simulink model "test_fastterminal_formation_gazebo_paper_cts23a"  (R2023a)
settings: Solver=FixedStepAuto  StartTime=0.0  StopTime=inf  RelTol=1e-3
undefined symbols (not defined in the file or in its folder): angular, DiscIntNeverNeededParam, linear
libraries: ros2lib x11, simulink x4, robotcorelib x4
(part 1 of 2)
settings Model: Creator=johvany  LastModifiedBy=l15
settings OptimizationCC: EnhancedBackFolding=on  PassReuseOutputArgsThreshold=0  MaxStackSize=64  OptimizeBlockOrder=speed  DifferentSizesBufferReuse=on  OptimizationCustomize=off
settings DebuggingCC: ParameterTunabilityLossMsg=error
settings HardwareCC: ProdBitPerLong=64  ProdHWDeviceType=Intel->x86-64 (Linux 64)  UseEmbeddedCoderFeatures=off
settings SFSimCC: MATLABDynamicMemAlloc=off
settings RTWCC: Description=Simulink Desktop Real-Time  SystemTargetFile=sldrt.tlc  TemplateMakefile=sldrt.tmf  Toolchain=Colcon Tools  RTWCompilerOptimization=on
settings CodeAppCC: ForceParamTrailComments=on  MaxIdLength=95  OperatorAnnotations=on
settings SimulinkDesktopRealTimeCC: TargetLibSuffix=_sldrt.a  TargetPreCompLibLocation=/usr/local/MATLAB/R2023b/toolbox/sldrt/lib/glnxa64  TargetLangStandard=C89/C90 (ANSI)

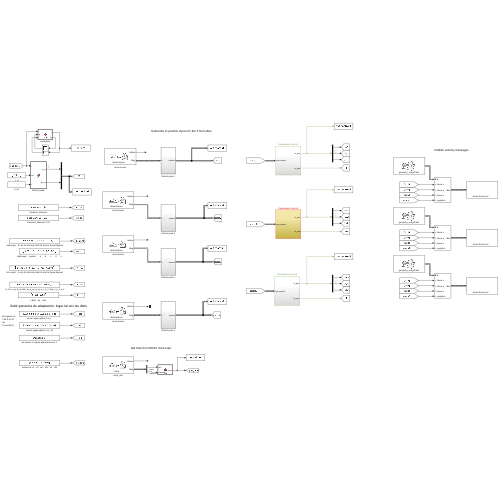
[thumbnail: Simulink's stored preview of the top-level diagram]
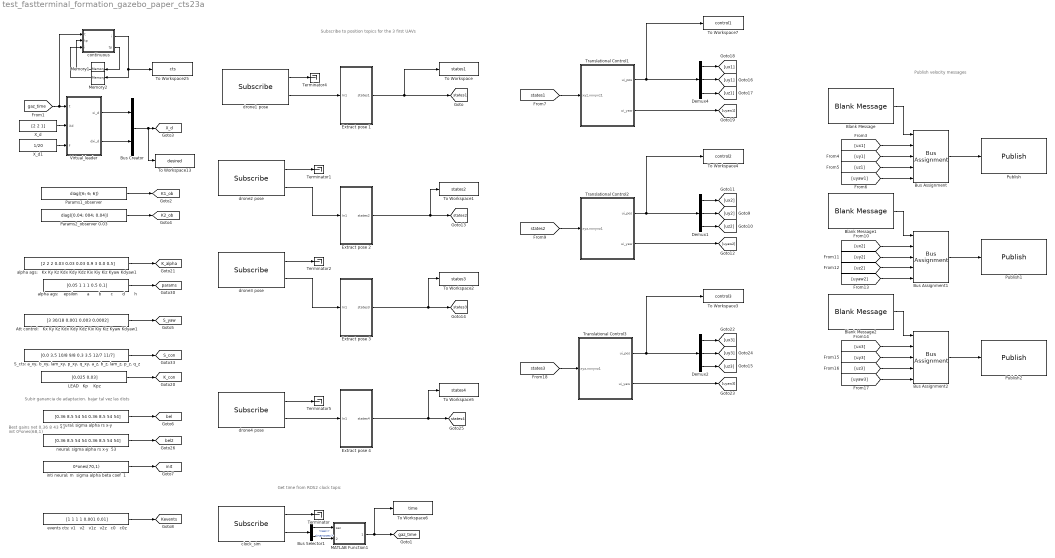
== system test_fastterminal_formation_gazebo_paper_cts23a ==
  note: Subir ganancia de adaptacion. bajar tal vez las dists
  note: Publish velocity messages
  note: Subscribe to position topics for the 3 first UAVs
  note: Get time from ROS2 clock topic
  note: Best gains net
      | 0.36 8 43 43
      | init
      | 0*ones(68,1)
  Att control:   Kx Ky Kz Kdx Kdy Kdz Kix Kiy Kiz Kyaw Kdyaw1 : Constant  Value=[3 30/18 0.001 0.003 0.0002]
  Blank Message : ros2lib/Blank Message  messageClass=Message  entityType=geometry_msgs/Twist  messageType=geometry_msgs/Twist  SampleTime=inf
  Blank Message1 : ros2lib/Blank Message  messageClass=Message  entityType=geometry_msgs/Twist  messageType=geometry_msgs/Twist  SampleTime=inf
  Blank Message2 : ros2lib/Blank Message  messageClass=Message  entityType=geometry_msgs/Twist  messageType=geometry_msgs/Twist  SampleTime=inf
  Bus Assignment : BusAssignment  AssignedSignals=linear.x,linear.y,linear.z,angular.z
  Bus Assignment1 : BusAssignment  AssignedSignals=linear.x,linear.y,linear.z,angular.z
  Bus Assignment2 : BusAssignment  AssignedSignals=linear.x,linear.y,linear.z,angular.z
  Bus Creator : BusCreator  Inputs=2
  Bus Selector1 : BusSelector  OutputSignals=clock.sec,clock.nanosec
  Demux1 : Demux  Outputs=3
  Demux2 : Demux  Outputs=3
  Demux4 : Demux  Outputs=3
  Extract pose 1 : Subsystem
  Extract pose 2 : Subsystem
  Extract pose 3 : Subsystem
  Extract pose 4 : Subsystem
  LEAD   Kp    Kpz : Constant  Value=[0.025 0.03]
  MATLAB Function1 : MATLAB Function  TreatAsAtomicUnit=on
  Memory1 : Memory
  Memory2 : Memory
  Params1_observer : Constant  Value=diag([6; 6; 6])
  Params2_observer 0.03 : Constant  Value=diag([0.04; 004; 0.04])
  Publish : ros2lib/Publish  topicSource=Select from ROS network  topic=/drone1/cmd_vel  messageType=geometry_msgs/Twist  QOSHistory=Keep last  QOSDepth=1  QOSReliability=Reliable  QOSDurability=Volatile
  Publish1 : ros2lib/Publish  topicSource=Select from ROS network  topic=/drone2/cmd_vel  messageType=geometry_msgs/Twist  QOSHistory=Keep last  QOSDepth=1  QOSReliability=Reliable  QOSDurability=Volatile
  Publish2 : ros2lib/Publish  topicSource=Select from ROS network  topic=/drone3/cmd_vel  messageType=geometry_msgs/Twist  QOSHistory=Keep last  QOSDepth=1  QOSReliability=Reliable  QOSDurability=Volatile
  "S_cts: a_xy, b_xy, lam_xy, p_xy, q_xy, a_z, b_z, lam_z, p_z, q_z" : Constant  Value=[0.0 3.5 10/8 9/8 0.3 3.5 12/7 11/7]
  Terminator{,1..2,4..5} (5 alike) : Terminator
  To Workspace : ToWorkspace  VariableName=states1  SampleTime=-1
  To Workspace1 : ToWorkspace  VariableName=states2  SampleTime=-1
  To Workspace13 : ToWorkspace  VariableName=desired  SampleTime=-1
  To Workspace2 : ToWorkspace  VariableName=states3  SampleTime=-1
  To Workspace25 : ToWorkspace  VariableName=cts  SampleTime=-1
  To Workspace3 : ToWorkspace  VariableName=control3  SampleTime=-1
  To Workspace4 : ToWorkspace  VariableName=control2  SampleTime=-1
  To Workspace5 : ToWorkspace  VariableName=states4  SampleTime=-1
  To Workspace6 : ToWorkspace  VariableName=time  SampleTime=-1
  To Workspace7 : ToWorkspace  VariableName=control1  SampleTime=-1
  Translational Control1 : Subsystem
  Translational Control2 : Subsystem
  Translational Control3 : Subsystem
  Virtual_leader : MATLAB Function  TreatAsAtomicUnit=on
  X_d : Constant  Value=[2 2 1]
  X_d1 : Constant  Value=1/20
  alpha ags:    epsilon       a       b       c       d       h : Constant  Value=[0.05 1 1 1 0.5 0.1]
  alpha ags:   Kx Ky Kz Kdx Kdy Kdz Kix Kiy Kiz Kyaw Kdyaw1 : Constant  Value=[2 2 2 0.03 0.03 0.03 0.9 3 0.0 0.5]
  clock_sim : ros2lib/Subscribe  topicSource=Select from ROS network  topic=/clock  messageType=rosgraph_msgs/Clock  sampleTime=-1  QOSHistory=Keep last  QOSDepth=1  QOSReliability=Reliable  QOSDurability=Volatile
  continuous : MATLAB Function  TreatAsAtomicUnit=on
  drone1 pose : ros2lib/Subscribe  topicSource=Select from ROS network  topic=/drone1/pose  messageType=geometry_msgs/PoseStamped  sampleTime=-1  QOSHistory=Keep last  QOSDepth=1  QOSReliability=Reliable  QOSDurability=Volatile
  drone2 pose : ros2lib/Subscribe  topicSource=Select from ROS network  topic=/drone2/pose  messageType=geometry_msgs/PoseStamped  sampleTime=-1  QOSHistory=Keep last  QOSDepth=1  QOSReliability=Reliable  QOSDurability=Volatile
  drone3 pose : ros2lib/Subscribe  topicSource=Select from ROS network  topic=/drone3/pose  messageType=geometry_msgs/PoseStamped  sampleTime=-1  QOSHistory=Keep last  QOSDepth=1  QOSReliability=Reliable  QOSDurability=Volatile
  drone4 pose : ros2lib/Subscribe  topicSource=Select from ROS network  topic=/drone4/pose  messageType=geometry_msgs/PoseStamped  sampleTime=-1  QOSHistory=Keep last  QOSDepth=1  QOSReliability=Reliable  QOSDurability=Volatile
  events cts: v1   v2   v1z   v2z   c0   c0z : Constant  Value=[1 1 1 1 0.001 0.01]
  inti neural: m  sigma alpha beta coef  1 : Constant  Value=0*ones(70,1)
  "neural: sigma alpha rs x-y  " : Constant  Value=[0.36 8.5 54 54 0.36 8.5 54 54]
  neural: sigma alpha rs x-y  53 : Constant  Value=[0.36 8.5 54 54 0.36 8.5 54 54]
  tag scope: K1_ob=global, K2_ob=global, K_alpha=global, K_con=global, Kevents=global, S_con=global, S_yaw=global, X_d=global, bel2=global, bel=global, gaz_time=global, init=global, params=global, states1=global, states2=global, states3=global, states4=global
  wires:
  clock_sim/1 -> Terminator/1
  drone2 pose/2 -> Extract pose 2/1(In1)
  drone2 pose/1 -> Terminator1/1
  drone3 pose/2 -> Extract pose 3/1(In1)
  drone3 pose/1 -> Terminator2/1
  Blank Message/1 -> Bus Assignment/1
  Bus Assignment/1 -> Publish/1
  Blank Message1/1 -> Bus Assignment1/1
  Bus Assignment1/1 -> Publish1/1
  Blank Message2/1 -> Bus Assignment2/1
  Bus Assignment2/1 -> Publish2/1
  clock_sim/2 -> Bus Selector1/1
  Bus Selector1/1 -> MATLAB Function1/1(sec)  "<sec>"
  Bus Selector1/2 -> MATLAB Function1/2(nanosec)  "<nanosec>"
  Virtual_leader/2(dxi_d) -> Bus Creator/2
  Bus Creator/1 -> To Workspace13/1, [X_d]
  Virtual_leader/1(xi_d) -> Bus Creator/1
  drone1 pose/1 -> Terminator4/1
  drone1 pose/2 -> Extract pose 1/1(In1)
  MATLAB Function1/1(gaz_time) -> To Workspace6/1, [gaz_time]
  Extract pose 1/1(states1) -> To Workspace/1, [states1]
  [ux1] -> Bus Assignment/2
  [uy1] -> Bus Assignment/3
  [uz1] -> Bus Assignment/4
  [uyaw1] -> Bus Assignment/5
  X_d/1 -> Virtual_leader/2(Xd)
  Extract pose 2/1(states2) -> To Workspace1/1, [states2]
  Extract pose 3/1(states3) -> To Workspace2/1, [states3]
  [ux2] -> Bus Assignment1/2
  [uy2] -> Bus Assignment1/3
  [uz2] -> Bus Assignment1/4
  [uyaw2] -> Bus Assignment1/5
  [uy3] -> Bus Assignment2/3
  [uyaw3] -> Bus Assignment2/5
  [uz3] -> Bus Assignment2/4
  [ux3] -> Bus Assignment2/2
  Translational Control1/2(ui_yaw) -> [uyaw1]
  Demux4/2 -> [uy1]
  Demux4/3 -> [uz1]
  [states1] -> Translational Control1/1(xyz,vxvyvz1)
  Demux4/1 -> [ux1]
  LEAD   Kp    Kpz/1 -> [K_con]
  alpha ags:   Kx Ky Kz Kdx Kdy Kdz Kix Kiy Kiz Kyaw Kdyaw1/1 -> [K_alpha]
  alpha ags:    epsilon       a       b       c       d       h/1 -> [params]
  X_d1/1 -> Virtual_leader/3(f)
  "S_cts: a_xy, b_xy, lam_xy, p_xy, q_xy, a_z, b_z, lam_z, p_z, q_z"/1 -> [S_con]
  "neural: sigma alpha rs x-y  "/1 -> [bel]
  inti neural: m  sigma alpha beta coef  1/1 -> [init]
  Translational Control1/1(ui_pos) -> Demux4/1, To Workspace7/1
  Params1_observer/1 -> [K1_ob]
  Params2_observer 0.03/1 -> [K2_ob]
  events cts: v1   v2   v1z   v2z   c0   c0z/1 -> [Kevents]
  Translational Control2/1(ui_pos) -> Demux1/1, To Workspace4/1
  Demux1/1 -> [ux2]
  [states2] -> Translational Control2/1(xyz,vxvyvz1)
  Demux1/3 -> [uz2]
  Demux1/2 -> [uy2]
  Translational Control2/2(ui_yaw) -> [uyaw2]
  Translational Control3/2(ui_yaw) -> [uyaw3]
  Demux2/2 -> [uy3]
  Demux2/3 -> [uz3]
  [states3] -> Translational Control3/1(xyz,vxvyvz1)
  Demux2/1 -> [ux3]
  Translational Control3/1(ui_pos) -> Demux2/1, To Workspace3/1
  Extract pose 4/1(states4) -> [states4], To Workspace5/1
  drone4 pose/1 -> Terminator5/1
  drone4 pose/2 -> Extract pose 4/1(In1)
  neural: sigma alpha rs x-y  53/1 -> [bel2]
  Memory1/1 -> continuous/2("tp ")
  Memory2/1 -> continuous/3("i ")
  [gaz_time] -> continuous/1(t), Virtual_leader/1(t)
  continuous/1(i) -> To Workspace25/1, Memory2/1
  continuous/2(tp) -> Memory1/1
  Att control:   Kx Ky Kz Kdx Kdy Kdz Kix Kiy Kiz Kyaw Kdyaw1/1 -> [S_yaw]

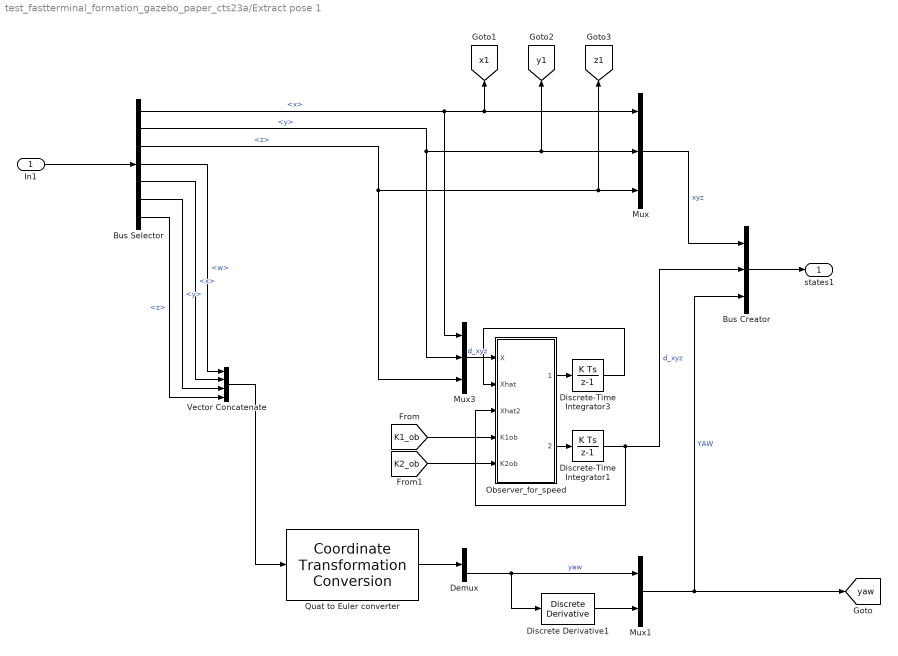
== system test_fastterminal_formation_gazebo_paper_cts23a/Extract pose 1 ==
  In1 : Inport
  Bus Creator : BusCreator  Inputs=3
  Bus Selector : BusSelector  OutputSignals=pose.position.x,pose.position.y,pose.position.z,pose.orientation.w,pose.orientation.x,pose.orientation.y,pose.orientation.z
  Demux : Demux  Outputs=3
  Discrete Derivative1 : simulink/Discrete/Discrete Derivative  gainval=1.0  ICPrevScaledInput=0.0  OutMin=[]  OutMax=[]  OutDataType=fixdt(1, 16)  OutScaling=2^-10  DoSatur=off
  Discrete-Time Integrator1 : DiscreteIntegrator  SampleTime=-1  UpperSaturationLimit=1  LowerSaturationLimit=-1  ICPrevOutput=DiscIntNeverNeededParam  ICPrevScaledInput=DiscIntNeverNeededParam
  Discrete-Time Integrator3 : DiscreteIntegrator  SampleTime=-1  UpperSaturationLimit=1  LowerSaturationLimit=-1  ICPrevOutput=DiscIntNeverNeededParam  ICPrevScaledInput=DiscIntNeverNeededParam
  Mux : Mux  Inputs=3
  Mux1 : Mux  Inputs=2
  Mux3 : Mux  Inputs=3
  Observer_for_speed : MATLAB Function  TreatAsAtomicUnit=on
  Quat to Euler converter : robotcorelib/Coordinate Transformation Conversion  InputRepresentation=Quaternion  InputEulerSequence=ZYX  ShowTrVecInputPort=on  OutputRepresentation=Euler Angles  OutputEulerSequence=XYZ  ShowTrVecOutputPort=on  SimulateUsing=Interpreted execution
      settings: LibrarySourceBlock=roslib/Utilities/Coordinate Transformation Conversion
  Vector Concatenate : Concatenate  NumInputs=4
  states1 : Outport
  tag scope: x1=global, y1=global, yaw=global, z1=global
  wires:
  Bus Selector/5 -> Vector Concatenate/2  "<x>"
  Quat to Euler converter/1 -> Demux/1
  Bus Selector/6 -> Vector Concatenate/3  "<y>"
  Bus Selector/7 -> Vector Concatenate/4  "<z>"
  Vector Concatenate/1 -> Quat to Euler converter/1
  In1/1 -> Bus Selector/1
  Bus Selector/4 -> Vector Concatenate/1  "<w>"
  Demux/3 -> Discrete Derivative1/1, Mux1/1  "yaw"
  Mux/1 -> Bus Creator/1  "xyz"
  Bus Creator/1 -> states1/1
  Discrete Derivative1/1 -> Mux1/2
  Bus Selector/3 -> Mux3/3, [z1], Mux/3  "<z>"
  Bus Selector/2 -> Mux3/2, [y1], Mux/2  "<y>"
  Bus Selector/1 -> Mux3/1, [x1], Mux/1  "<x>"
  Mux1/1 -> [yaw], Bus Creator/3  "YAW"
  Discrete-Time Integrator1/1 -> Observer_for_speed/3(Xhat2), Bus Creator/2  "d_xyz"
  Discrete-Time Integrator3/1 -> Observer_for_speed/2(Xhat)
  Observer_for_speed/1(dXhat_1) -> Discrete-Time Integrator3/1
  Observer_for_speed/2(dXhat_2) -> Discrete-Time Integrator1/1
  Mux3/1 -> Observer_for_speed/1(X)  "d_xyz"
  [K1_ob] -> Observer_for_speed/4(K1ob)
  [K2_ob] -> Observer_for_speed/5(K2ob)

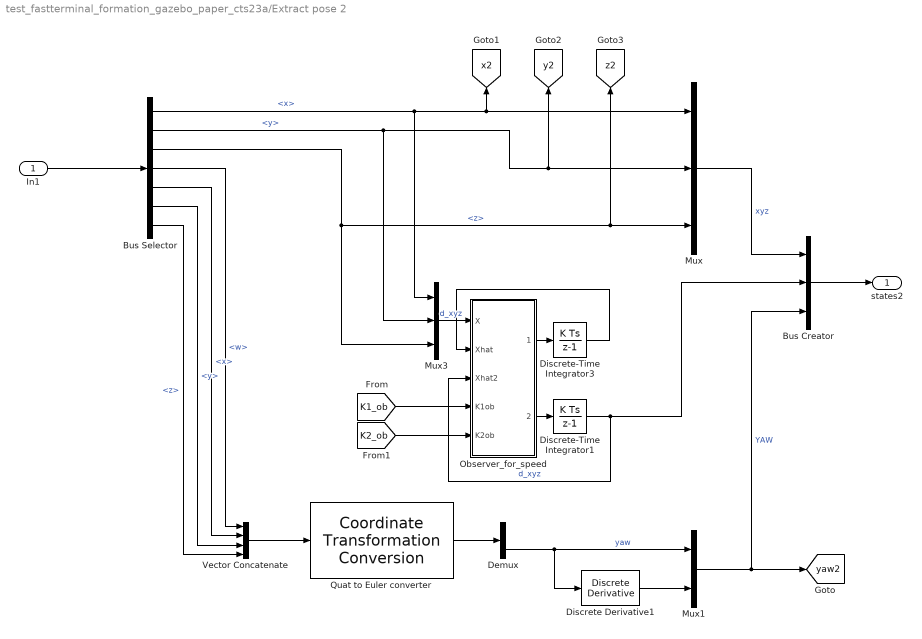
== system test_fastterminal_formation_gazebo_paper_cts23a/Extract pose 2 ==
  In1 : Inport
  Bus Creator : BusCreator  Inputs=3
  Bus Selector : BusSelector  OutputSignals=pose.position.x,pose.position.y,pose.position.z,pose.orientation.w,pose.orientation.x,pose.orientation.y,pose.orientation.z
  Demux : Demux  Outputs=3
  Discrete Derivative1 : simulink/Discrete/Discrete Derivative  gainval=1.0  ICPrevScaledInput=0.0  OutMin=[]  OutMax=[]  OutDataType=fixdt(1, 16)  OutScaling=2^-10  DoSatur=off
  Discrete-Time Integrator1 : DiscreteIntegrator  SampleTime=-1  UpperSaturationLimit=1  LowerSaturationLimit=-1  ICPrevOutput=DiscIntNeverNeededParam  ICPrevScaledInput=DiscIntNeverNeededParam
  Discrete-Time Integrator3 : DiscreteIntegrator  SampleTime=-1  UpperSaturationLimit=1  LowerSaturationLimit=-1  ICPrevOutput=DiscIntNeverNeededParam  ICPrevScaledInput=DiscIntNeverNeededParam
  Mux : Mux  Inputs=3
  Mux1 : Mux  Inputs=2
  Mux3 : Mux  Inputs=3
  Observer_for_speed : MATLAB Function  TreatAsAtomicUnit=on
  Quat to Euler converter : robotcorelib/Coordinate Transformation Conversion  InputRepresentation=Quaternion  InputEulerSequence=ZYX  ShowTrVecInputPort=on  OutputRepresentation=Euler Angles  OutputEulerSequence=XYZ  ShowTrVecOutputPort=on  SimulateUsing=Interpreted execution
      settings: LibrarySourceBlock=roslib/Utilities/Coordinate Transformation Conversion
  Vector Concatenate : Concatenate  NumInputs=4
  states2 : Outport
  tag scope: x2=global, y2=global, yaw2=global, z2=global
  wires:
  Discrete Derivative1/1 -> Mux1/2
  Bus Creator/1 -> states2/1
  Mux/1 -> Bus Creator/1  "xyz"
  Demux/3 -> Discrete Derivative1/1, Mux1/1  "yaw"
  Bus Selector/4 -> Vector Concatenate/1  "<w>"
  In1/1 -> Bus Selector/1
  Vector Concatenate/1 -> Quat to Euler converter/1
  Bus Selector/7 -> Vector Concatenate/4  "<z>"
  Bus Selector/6 -> Vector Concatenate/3  "<y>"
  Quat to Euler converter/1 -> Demux/1
  Bus Selector/5 -> Vector Concatenate/2  "<x>"
  Mux3/1 -> Observer_for_speed/1(X)  "d_xyz"
  Observer_for_speed/1(dXhat_1) -> Discrete-Time Integrator3/1
  Observer_for_speed/2(dXhat_2) -> Discrete-Time Integrator1/1
  [K1_ob] -> Observer_for_speed/4(K1ob)
  Bus Selector/2 -> Mux3/2, [y2], Mux/2  "<y>"
  Bus Selector/1 -> Mux3/1, [x2], Mux/1  "<x>"
  Discrete-Time Integrator3/1 -> Observer_for_speed/2(Xhat)
  Discrete-Time Integrator1/1 -> Bus Creator/2, Observer_for_speed/3(Xhat2)  "d_xyz"
  [K2_ob] -> Observer_for_speed/5(K2ob)
  Bus Selector/3 -> Mux3/3, [z2], Mux/3  "<z>"
  Mux1/1 -> [yaw2], Bus Creator/3  "YAW"

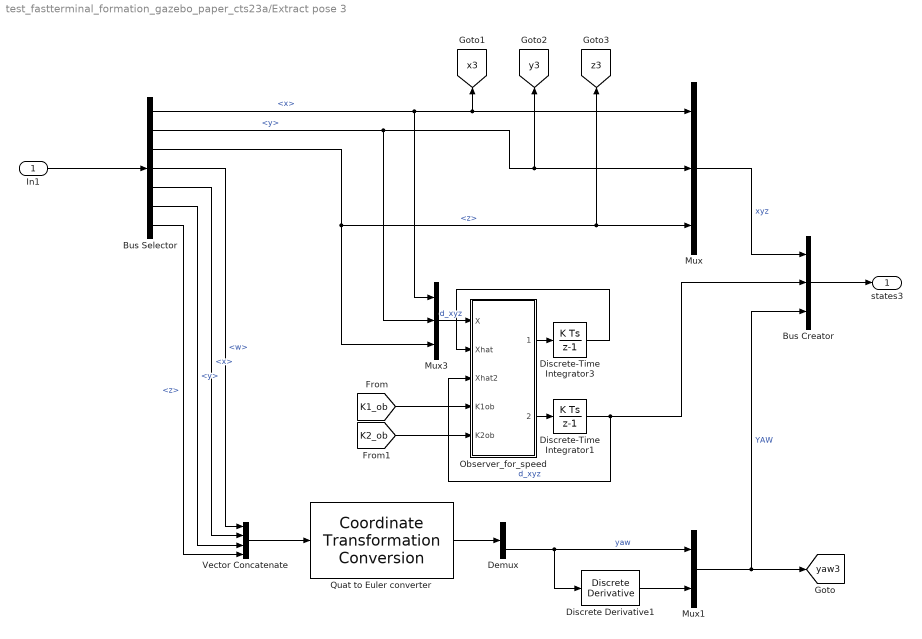
== system test_fastterminal_formation_gazebo_paper_cts23a/Extract pose 3 ==
  In1 : Inport
  Bus Creator : BusCreator  Inputs=3
  Bus Selector : BusSelector  OutputSignals=pose.position.x,pose.position.y,pose.position.z,pose.orientation.w,pose.orientation.x,pose.orientation.y,pose.orientation.z
  Demux : Demux  Outputs=3
  Discrete Derivative1 : simulink/Discrete/Discrete Derivative  gainval=1.0  ICPrevScaledInput=0.0  OutMin=[]  OutMax=[]  OutDataType=fixdt(1, 16)  OutScaling=2^-10  DoSatur=off
  Discrete-Time Integrator1 : DiscreteIntegrator  SampleTime=-1  UpperSaturationLimit=1  LowerSaturationLimit=-1  ICPrevOutput=DiscIntNeverNeededParam  ICPrevScaledInput=DiscIntNeverNeededParam
  Discrete-Time Integrator3 : DiscreteIntegrator  SampleTime=-1  UpperSaturationLimit=1  LowerSaturationLimit=-1  ICPrevOutput=DiscIntNeverNeededParam  ICPrevScaledInput=DiscIntNeverNeededParam
  Mux : Mux  Inputs=3
  Mux1 : Mux  Inputs=2
  Mux3 : Mux  Inputs=3
  Observer_for_speed : MATLAB Function  TreatAsAtomicUnit=on
  Quat to Euler converter : robotcorelib/Coordinate Transformation Conversion  InputRepresentation=Quaternion  InputEulerSequence=ZYX  ShowTrVecInputPort=on  OutputRepresentation=Euler Angles  OutputEulerSequence=XYZ  ShowTrVecOutputPort=on  SimulateUsing=Interpreted execution
      settings: LibrarySourceBlock=roslib/Utilities/Coordinate Transformation Conversion
  Vector Concatenate : Concatenate  NumInputs=4
  states3 : Outport
  tag scope: x3=global, y3=global, yaw3=global, z3=global
  wires:
  Mux1/1 -> Bus Creator/3, [yaw3]  "YAW"
  Bus Selector/3 -> [z3], Mux/3, Mux3/3  "<z>"
  [K2_ob] -> Observer_for_speed/5(K2ob)
  Discrete-Time Integrator1/1 -> Observer_for_speed/3(Xhat2), Bus Creator/2  "d_xyz"
  Discrete-Time Integrator3/1 -> Observer_for_speed/2(Xhat)
  Bus Selector/1 -> [x3], Mux/1, Mux3/1  "<x>"
  Bus Selector/2 -> [y3], Mux/2, Mux3/2  "<y>"
  [K1_ob] -> Observer_for_speed/4(K1ob)
  Observer_for_speed/2(dXhat_2) -> Discrete-Time Integrator1/1
  Observer_for_speed/1(dXhat_1) -> Discrete-Time Integrator3/1
  Mux3/1 -> Observer_for_speed/1(X)  "d_xyz"
  Bus Selector/5 -> Vector Concatenate/2  "<x>"
  Quat to Euler converter/1 -> Demux/1
  Bus Selector/6 -> Vector Concatenate/3  "<y>"
  Bus Selector/7 -> Vector Concatenate/4  "<z>"
  Vector Concatenate/1 -> Quat to Euler converter/1
  In1/1 -> Bus Selector/1
  Bus Selector/4 -> Vector Concatenate/1  "<w>"
  Demux/3 -> Mux1/1, Discrete Derivative1/1  "yaw"
  Mux/1 -> Bus Creator/1  "xyz"
  Bus Creator/1 -> states3/1
  Discrete Derivative1/1 -> Mux1/2

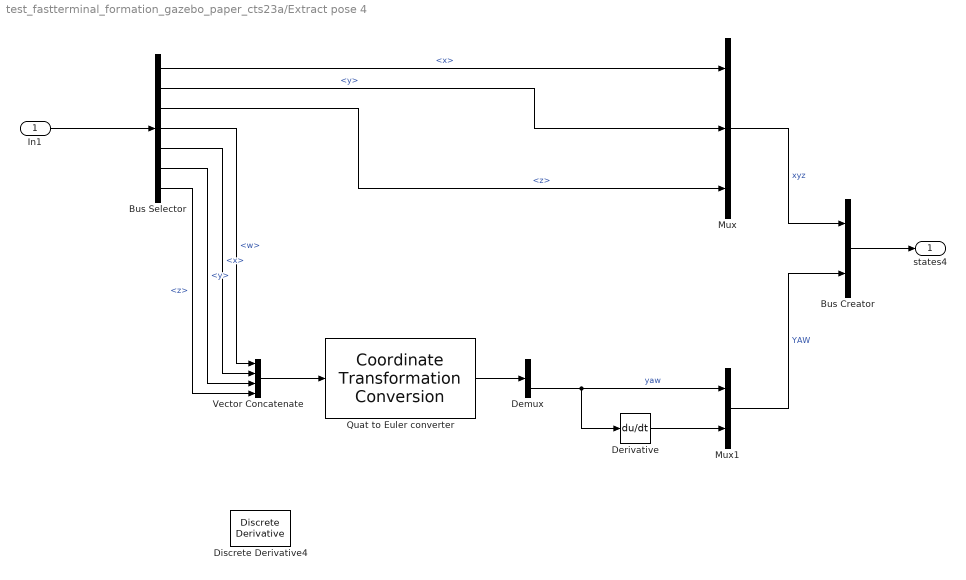
== system test_fastterminal_formation_gazebo_paper_cts23a/Extract pose 4 ==
  In1 : Inport
  Bus Creator : BusCreator  Inputs=2
  Bus Selector : BusSelector  OutputSignals=pose.position.x,pose.position.y,pose.position.z,pose.orientation.w,pose.orientation.x,pose.orientation.y,pose.orientation.z
  Demux : Demux  Outputs=3
  Derivative : Derivative
  Discrete Derivative4 : simulink/Discrete/Discrete Derivative  gainval=1.0  ICPrevScaledInput=0.0  OutMin=[]  OutMax=[]  OutDataType=fixdt(1, 16)  OutScaling=2^-10  DoSatur=off
  Mux : Mux  Inputs=3
  Mux1 : Mux  Inputs=2
  Quat to Euler converter : robotcorelib/Coordinate Transformation Conversion  InputRepresentation=Quaternion  InputEulerSequence=ZYX  ShowTrVecInputPort=on  OutputRepresentation=Euler Angles  OutputEulerSequence=XYZ  ShowTrVecOutputPort=on  SimulateUsing=Interpreted execution
      settings: LibrarySourceBlock=roslib/Utilities/Coordinate Transformation Conversion
  Vector Concatenate : Concatenate  NumInputs=4
  states4 : Outport
  wires:
  Bus Selector/5 -> Vector Concatenate/2  "<x>"
  Quat to Euler converter/1 -> Demux/1
  Bus Selector/6 -> Vector Concatenate/3  "<y>"
  Bus Selector/1 -> Mux/1  "<x>"
  Bus Selector/7 -> Vector Concatenate/4  "<z>"
  Vector Concatenate/1 -> Quat to Euler converter/1
  In1/1 -> Bus Selector/1
  Bus Selector/4 -> Vector Concatenate/1  "<w>"
  Bus Selector/2 -> Mux/2  "<y>"
  Bus Selector/3 -> Mux/3  "<z>"
  Demux/3 -> Derivative/1, Mux1/1  "yaw"
  Mux/1 -> Bus Creator/1  "xyz"
  Bus Creator/1 -> states4/1
  Derivative/1 -> Mux1/2
  Mux1/1 -> Bus Creator/2  "YAW"

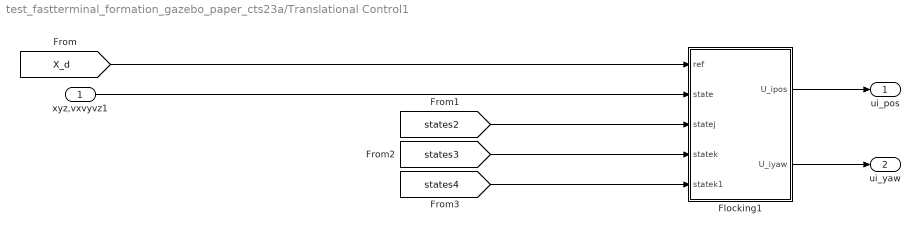
== system test_fastterminal_formation_gazebo_paper_cts23a/Translational Control1 ==
  xyz,vxvyvz1 : Inport
  Flocking1 : Subsystem
  ui_pos : Outport  VectorParamsAs1DForOutWhenUnconnected=off
  ui_yaw : Outport  Port=2  VectorParamsAs1DForOutWhenUnconnected=off
  wires:
  [states2] -> Flocking1/3(statej)
  [states3] -> Flocking1/4(statek)
  [states4] -> Flocking1/5(statek1)
  Flocking1/1(U_ipos) -> ui_pos/1
  Flocking1/2(U_iyaw) -> ui_yaw/1
  [X_d] -> Flocking1/1(ref)
  xyz,vxvyvz1/1 -> Flocking1/2(state)

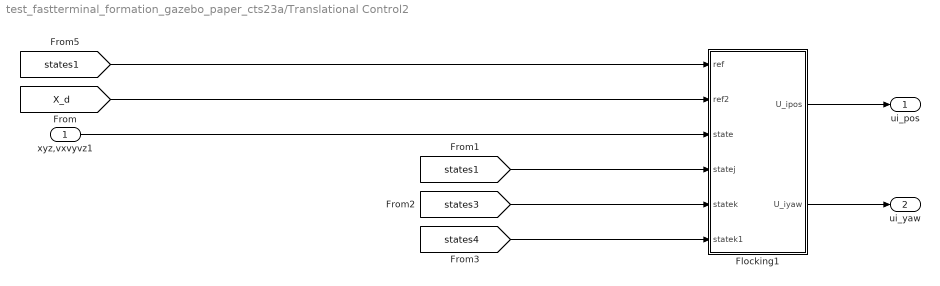
== system test_fastterminal_formation_gazebo_paper_cts23a/Translational Control2 ==
  xyz,vxvyvz1 : Inport
  Flocking1 : Subsystem
  ui_pos : Outport  VectorParamsAs1DForOutWhenUnconnected=off
  ui_yaw : Outport  Port=2  VectorParamsAs1DForOutWhenUnconnected=off
  wires:
  Flocking1/2(U_iyaw) -> ui_yaw/1
  Flocking1/1(U_ipos) -> ui_pos/1
  [states4] -> Flocking1/6(statek1)
  [states3] -> Flocking1/5(statek)
  [states1] -> Flocking1/4(statej)
  [states1] -> Flocking1/1(ref)
  [X_d] -> Flocking1/2(ref2)
  xyz,vxvyvz1/1 -> Flocking1/3(state)

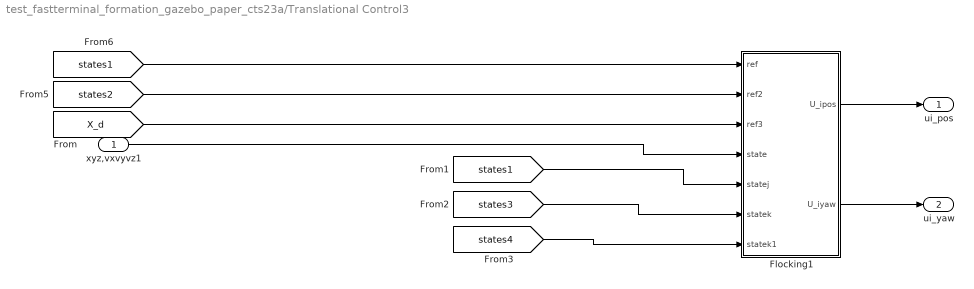
== system test_fastterminal_formation_gazebo_paper_cts23a/Translational Control3 ==
  xyz,vxvyvz1 : Inport
  Flocking1 : Subsystem
  ui_pos : Outport  VectorParamsAs1DForOutWhenUnconnected=off
  ui_yaw : Outport  Port=2  VectorParamsAs1DForOutWhenUnconnected=off
  wires:
  [states1] -> Flocking1/5(statej)
  [states3] -> Flocking1/6(statek)
  [states4] -> Flocking1/7(statek1)
  Flocking1/1(U_ipos) -> ui_pos/1
  Flocking1/2(U_iyaw) -> ui_yaw/1
  [states1] -> Flocking1/1(ref)
  [states2] -> Flocking1/2(ref2)
  [X_d] -> Flocking1/3(ref3)
  xyz,vxvyvz1/1 -> Flocking1/4(state)

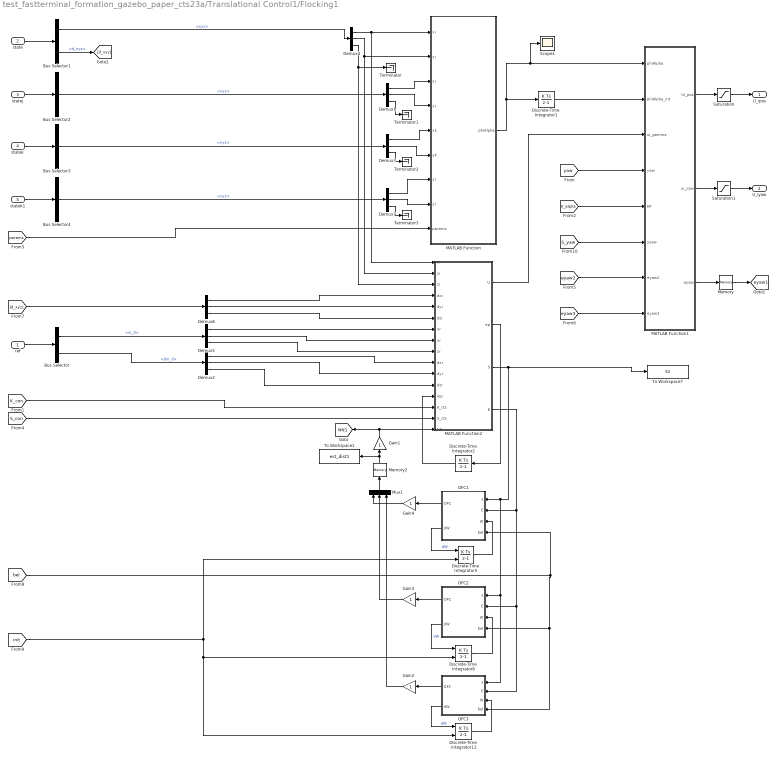
== system test_fastterminal_formation_gazebo_paper_cts23a/Translational Control1/Flocking1 ==
  ref : Inport
  state : Inport  Port=2
  statej : Inport  Port=3
  statek : Inport  Port=4
  statek1 : Inport  Port=5
  Bus Selector : BusSelector  OutputSignals=xi_d,dxi_d
  Bus Selector1 : BusSelector  OutputSignals=xyz,d_xyz
  Bus Selector2 : BusSelector  OutputSignals=xyz
  Bus Selector3 : BusSelector  OutputSignals=xyz
  Bus Selector4 : BusSelector  OutputSignals=xyz
  Demux{1..7} (7 alike) : Demux  Outputs=3
  Discrete-Time Integrator1 : DiscreteIntegrator  SampleTime=-1  LimitOutput=on  UpperSaturationLimit=5  LowerSaturationLimit=-5  ICPrevOutput=DiscIntNeverNeededParam  ICPrevScaledInput=DiscIntNeverNeededParam
  Discrete-Time Integrator12 : DiscreteIntegrator  InitialConditionSource=external  SampleTime=-1  UpperSaturationLimit=0.15  LowerSaturationLimit=-0.15  ICPrevOutput=DiscIntNeverNeededParam  ICPrevScaledInput=DiscIntNeverNeededParam
  Discrete-Time Integrator2 : DiscreteIntegrator  SampleTime=-1  LimitOutput=on  UpperSaturationLimit=2  LowerSaturationLimit=-2  ICPrevOutput=DiscIntNeverNeededParam  ICPrevScaledInput=DiscIntNeverNeededParam
  Discrete-Time Integrator5 : DiscreteIntegrator  InitialConditionSource=external  InitialCondition=0.25*ones(6,1)  SampleTime=-1  UpperSaturationLimit=0.15  LowerSaturationLimit=-0.15  ICPrevOutput=DiscIntNeverNeededParam  ICPrevScaledInput=DiscIntNeverNeededParam
  Discrete-Time Integrator8 : DiscreteIntegrator  InitialConditionSource=external  InitialCondition=0.25*ones(6,1)  SampleTime=-1  UpperSaturationLimit=0.15  LowerSaturationLimit=-0.15  ICPrevOutput=DiscIntNeverNeededParam  ICPrevScaledInput=DiscIntNeverNeededParam
  Gain{1..4} (4 alike) : Gain
  MATLAB Function : MATLAB Function  TreatAsAtomicUnit=on
  MATLAB Function1 : MATLAB Function  TreatAsAtomicUnit=on
  MATLAB Function2 : MATLAB Function  TreatAsAtomicUnit=on
  Memory : Memory
  Memory2 : Memory
  Mux1 : Mux  Inputs=3
  OFC1 : MATLAB Function  TreatAsAtomicUnit=on
  OFC2 : MATLAB Function  TreatAsAtomicUnit=on
  OFC3 : MATLAB Function  TreatAsAtomicUnit=on
  Saturation : Saturate  UpperLimit=1  LowerLimit=-1
  Saturation1 : Saturate  UpperLimit=1  LowerLimit=-1
  Scope1 : Scope
  Terminator{,1..3} (4 alike) : Terminator
  To Workspace1 : ToWorkspace  VariableName=est_dist1  SampleTime=-1
  To Workspace7 : ToWorkspace  VariableName=S1  SampleTime=-1
  U_ipos : Outport  VectorParamsAs1DForOutWhenUnconnected=off
  U_iyaw : Outport  Port=2  VectorParamsAs1DForOutWhenUnconnected=off
  tag scope: NN1=global, eyaw1=global
  wires:
  ref/1 -> Bus Selector/1
  state/1 -> Bus Selector1/1
  Bus Selector/1 -> Demux5/1  "<xi_d>"
  statej/1 -> Bus Selector2/1
  Bus Selector2/1 -> Demux1/1  "<xyz>"
  Demux4/1 -> MATLAB Function2/1(xi), MATLAB Function/1(xi)
  Demux4/2 -> MATLAB Function2/2(yi), MATLAB Function/2(yi)
  Demux1/1 -> MATLAB Function/3(xj)
  Demux1/2 -> MATLAB Function/4(yj)
  Discrete-Time Integrator1/1 -> MATLAB Function1/2(phiAlpha_int)
  MATLAB Function2/1(U) -> MATLAB Function1/3(ui_gamma)
  statek/1 -> Bus Selector3/1
  Demux3/1 -> MATLAB Function/5(xk)
  Demux3/2 -> MATLAB Function/6(yk)
  Bus Selector3/1 -> Demux3/1  "<xyz>"
  MATLAB Function/1(phiAlpha) -> Scope1/1, MATLAB Function1/1(phiAlpha), Discrete-Time Integrator1/1
  Demux5/1 -> MATLAB Function2/7(xr)
  Demux5/2 -> MATLAB Function2/8(yr)
  Demux4/3 -> Terminator/1, MATLAB Function2/3(zi)
  Demux3/3 -> Terminator2/1
  Demux5/3 -> MATLAB Function2/9(zr)
  MATLAB Function1/1(Ui_pos) -> Saturation/1
  Demux1/3 -> Terminator1/1
  statek1/1 -> Bus Selector4/1
  Demux7/1 -> MATLAB Function/7(xl)
  Demux7/2 -> MATLAB Function/8(yl)
  Demux7/3 -> Terminator3/1
  Bus Selector4/1 -> Demux7/1  "<xyz>"
  Bus Selector1/1 -> Demux4/1  "<xyz>"
  [yaw] -> MATLAB Function1/4(yaw)
  MATLAB Function1/2(ui_yaw) -> Saturation1/1
  MATLAB Function2/2(ep) -> Discrete-Time Integrator2/1
  Discrete-Time Integrator2/1 -> MATLAB Function2/13(iep)
  [K_con] -> MATLAB Function2/14(K_cts)
  MATLAB Function1/3(eyaw) -> Memory/1
  [K_alpha] -> MATLAB Function1/5(KP)
  [params] -> MATLAB Function/9(params)
  [S_con] -> MATLAB Function2/15(S_cts)
  Bus Selector/2 -> Demux2/1  "<dxi_d>"
  Demux2/1 -> MATLAB Function2/10(dxr)
  Demux2/2 -> MATLAB Function2/11(dyr)
  Demux2/3 -> MATLAB Function2/12(dzr)
  [eyaw2] -> MATLAB Function1/7(eyaw2)
  [eyaw3] -> MATLAB Function1/8(eyaw3)
  Memory/1 -> [eyaw1]
  MATLAB Function2/3(S) -> To Workspace7/1, OFC3/1(s), OFC2/1(s), OFC1/1(s)
  OFC3/1(OFC) -> Gain2/1
  OFC1/1(OFC) -> Gain4/1
  OFC2/1(OFC) -> Gain3/1
  OFC1/2(dW) -> Discrete-Time Integrator5/1  "dW"
  MATLAB Function2/4(E) -> OFC1/2(E), OFC3/2(E), OFC2/2(E)
  [bel] -> OFC3/4(bel), OFC2/4(bel), OFC1/4(bel)
  [init] -> Discrete-Time Integrator12/2, Discrete-Time Integrator8/2, Discrete-Time Integrator5/2
  OFC3/2(dW) -> Discrete-Time Integrator12/1  "dW"
  Discrete-Time Integrator12/1 -> OFC3/3(W)
  Gain3/1 -> Mux1/2
  Discrete-Time Integrator8/1 -> OFC2/3(W)
  Gain2/1 -> Mux1/3
  OFC2/2(dW) -> Discrete-Time Integrator8/1  "dW"
  Gain4/1 -> Mux1/1
  Gain1/1 -> [NN1], MATLAB Function2/16(NN)
  Saturation/1 -> U_ipos/1
  Saturation1/1 -> U_iyaw/1
  Discrete-Time Integrator5/1 -> OFC1/3(W)
  Mux1/1 -> Memory2/1
  Memory2/1 -> Gain1/1, To Workspace1/1
  Bus Selector1/2 -> [d_xyz]  "<d_xyz>"
  Demux6/1 -> MATLAB Function2/4(dxi)
  Demux6/2 -> MATLAB Function2/5(dyi)
  Demux6/3 -> MATLAB Function2/6(dzi)
  [d_xyz] -> Demux6/1
  [S_yaw] -> MATLAB Function1/6(syaw)

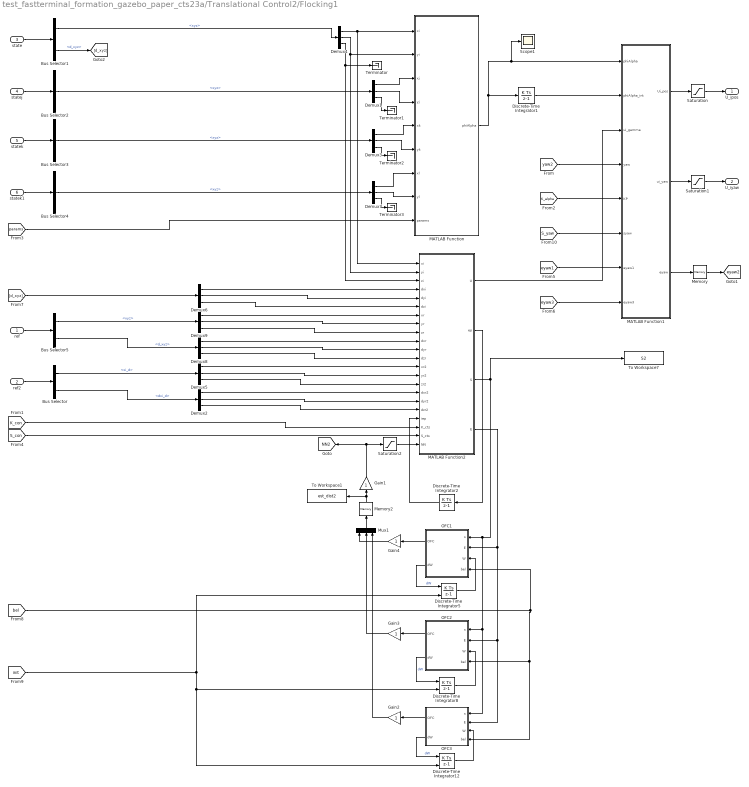
== system test_fastterminal_formation_gazebo_paper_cts23a/Translational Control2/Flocking1 ==
  ref : Inport
  ref2 : Inport  Port=2
  state : Inport  Port=3
  statej : Inport  Port=4
  statek : Inport  Port=5
  statek1 : Inport  Port=6
  Bus Selector : BusSelector  OutputSignals=xi_d,dxi_d
  Bus Selector1 : BusSelector  OutputSignals=xyz,d_xyz
  Bus Selector2 : BusSelector  OutputSignals=xyz
  Bus Selector3 : BusSelector  OutputSignals=xyz
  Bus Selector4 : BusSelector  OutputSignals=xyz
  Bus Selector5 : BusSelector  OutputSignals=xyz,d_xyz
  Demux{1..9} (9 alike) : Demux  Outputs=3
  Discrete-Time Integrator1 : DiscreteIntegrator  SampleTime=-1  LimitOutput=on  UpperSaturationLimit=5  LowerSaturationLimit=-5  ICPrevOutput=DiscIntNeverNeededParam  ICPrevScaledInput=DiscIntNeverNeededParam
  Discrete-Time Integrator12 : DiscreteIntegrator  InitialConditionSource=external  SampleTime=-1  UpperSaturationLimit=0.15  LowerSaturationLimit=-0.15  ICPrevOutput=DiscIntNeverNeededParam  ICPrevScaledInput=DiscIntNeverNeededParam
  Discrete-Time Integrator2 : DiscreteIntegrator  SampleTime=-1  LimitOutput=on  UpperSaturationLimit=2  LowerSaturationLimit=-2  ICPrevOutput=DiscIntNeverNeededParam  ICPrevScaledInput=DiscIntNeverNeededParam
  Discrete-Time Integrator5 : DiscreteIntegrator  InitialConditionSource=external  InitialCondition=0.25*ones(6,1)  SampleTime=-1  UpperSaturationLimit=0.15  LowerSaturationLimit=-0.15  ICPrevOutput=DiscIntNeverNeededParam  ICPrevScaledInput=DiscIntNeverNeededParam
  Discrete-Time Integrator8 : DiscreteIntegrator  InitialConditionSource=external  InitialCondition=0.25*ones(6,1)  SampleTime=-1  UpperSaturationLimit=0.15  LowerSaturationLimit=-0.15  ICPrevOutput=DiscIntNeverNeededParam  ICPrevScaledInput=DiscIntNeverNeededParam
  Gain{1..4} (4 alike) : Gain
  MATLAB Function : MATLAB Function  TreatAsAtomicUnit=on
  MATLAB Function1 : MATLAB Function  TreatAsAtomicUnit=on
  MATLAB Function2 : MATLAB Function  TreatAsAtomicUnit=on
  Memory : Memory
  Memory2 : Memory
  Mux1 : Mux  Inputs=3
  OFC1 : MATLAB Function  TreatAsAtomicUnit=on
  OFC2 : MATLAB Function  TreatAsAtomicUnit=on
  OFC3 : MATLAB Function  TreatAsAtomicUnit=on
  Saturation : Saturate  UpperLimit=1  LowerLimit=-1
  Saturation1 : Saturate  UpperLimit=1  LowerLimit=-1
  Saturation2 : Saturate  UpperLimit=0.9  LowerLimit=-0.9
  Scope1 : Scope
  Terminator{,1..3} (4 alike) : Terminator
  To Workspace1 : ToWorkspace  VariableName=est_dist2  SampleTime=-1
  To Workspace7 : ToWorkspace  VariableName=S2  SampleTime=-1
  U_ipos : Outport  VectorParamsAs1DForOutWhenUnconnected=off
  U_iyaw : Outport  Port=2  VectorParamsAs1DForOutWhenUnconnected=off
  tag scope: NN2=global, eyaw2=global
  wires:
  [d_xyz] -> Demux6/1
  Demux6/3 -> MATLAB Function2/6(dzi)
  Demux6/2 -> MATLAB Function2/5(dyi)
  Demux6/1 -> MATLAB Function2/4(dxi)
  Bus Selector1/2 -> [d_xyz]  "<d_xyz>"
  Memory2/1 -> To Workspace1/1, Gain1/1
  Mux1/1 -> Memory2/1
  Discrete-Time Integrator5/1 -> OFC1/3(W)
  Saturation1/1 -> U_iyaw/1
  Saturation/1 -> U_ipos/1
  Gain1/1 -> [NN2], Saturation2/1
  Gain4/1 -> Mux1/1
  OFC2/2(dW) -> Discrete-Time Integrator8/1  "dW"
  Gain2/1 -> Mux1/3
  Discrete-Time Integrator8/1 -> OFC2/3(W)
  Gain3/1 -> Mux1/2
  Discrete-Time Integrator12/1 -> OFC3/3(W)
  OFC3/2(dW) -> Discrete-Time Integrator12/1  "dW"
  [init] -> Discrete-Time Integrator5/2, Discrete-Time Integrator8/2, Discrete-Time Integrator12/2
  [bel] -> OFC1/4(bel), OFC2/4(bel), OFC3/4(bel)
  MATLAB Function2/4(E) -> OFC2/2(E), OFC3/2(E), OFC1/2(E)
  OFC1/2(dW) -> Discrete-Time Integrator5/1  "dW"
  OFC2/1(OFC) -> Gain3/1
  OFC1/1(OFC) -> Gain4/1
  OFC3/1(OFC) -> Gain2/1
  MATLAB Function2/3(S) -> To Workspace7/1, OFC1/1(s), OFC2/1(s), OFC3/1(s)
  Memory/1 -> [eyaw2]
  [eyaw3] -> MATLAB Function1/8(eyaw3)
  [eyaw1] -> MATLAB Function1/7(eyaw1)
  Bus Selector/2 -> Demux2/1  "<dxi_d>"
  [S_con] -> MATLAB Function2/21(S_cts)
  [params] -> MATLAB Function/9(params)
  [K_alpha] -> MATLAB Function1/5(KP)
  MATLAB Function1/3(eyaw) -> Memory/1
  [K_con] -> MATLAB Function2/20(K_cts)
  Discrete-Time Integrator2/1 -> MATLAB Function2/19(iep)
  MATLAB Function2/2(ep) -> Discrete-Time Integrator2/1
  MATLAB Function1/2(ui_yaw) -> Saturation1/1
  [yaw2] -> MATLAB Function1/4(yaw)
  Bus Selector1/1 -> Demux4/1  "<xyz>"
  Bus Selector4/1 -> Demux7/1  "<xyz>"
  Demux7/3 -> Terminator3/1
  Demux7/2 -> MATLAB Function/8(yl)
  Demux7/1 -> MATLAB Function/7(xl)
  statek1/1 -> Bus Selector4/1
  Demux1/3 -> Terminator1/1
  MATLAB Function1/1(Ui_pos) -> Saturation/1
  Demux3/3 -> Terminator2/1
  Demux4/3 -> MATLAB Function2/3(zi), Terminator/1
  MATLAB Function/1(phiAlpha) -> Discrete-Time Integrator1/1, MATLAB Function1/1(phiAlpha), Scope1/1
  Bus Selector3/1 -> Demux3/1  "<xyz>"
  Demux3/2 -> MATLAB Function/6(yk)
  Demux3/1 -> MATLAB Function/5(xk)
  statek/1 -> Bus Selector3/1
  MATLAB Function2/1(U) -> MATLAB Function1/3(ui_gamma)
  Discrete-Time Integrator1/1 -> MATLAB Function1/2(phiAlpha_int)
  Demux1/2 -> MATLAB Function/4(yj)
  Demux1/1 -> MATLAB Function/3(xj)
  Demux4/2 -> MATLAB Function/2(yi), MATLAB Function2/2(yi)
  Demux4/1 -> MATLAB Function/1(xi), MATLAB Function2/1(xi)
  Bus Selector2/1 -> Demux1/1  "<xyz>"
  statej/1 -> Bus Selector2/1
  Bus Selector/1 -> Demux5/1  "<xi_d>"
  state/1 -> Bus Selector1/1
  ref2/1 -> Bus Selector/1
  ref/1 -> Bus Selector5/1
  Bus Selector5/1 -> Demux9/1  "<xyz>"
  Bus Selector5/2 -> Demux8/1  "<d_xyz>"
  Demux9/2 -> MATLAB Function2/8(yr)
  Demux8/2 -> MATLAB Function2/11(dyr)
  Demux9/1 -> MATLAB Function2/7(xr)
  Demux9/3 -> MATLAB Function2/9(zr)
  Demux8/1 -> MATLAB Function2/10(dxr)
  Demux8/3 -> MATLAB Function2/12(dzr)
  Demux5/3 -> MATLAB Function2/15(zr2)
  Demux2/3 -> MATLAB Function2/18(dzr2)
  Demux5/2 -> MATLAB Function2/14(yr2)
  Demux2/2 -> MATLAB Function2/17(dyr2)
  Demux5/1 -> MATLAB Function2/13(xr2)
  Demux2/1 -> MATLAB Function2/16(dxr2)
  Saturation2/1 -> MATLAB Function2/22(NN)
  [S_yaw] -> MATLAB Function1/6(syaw)

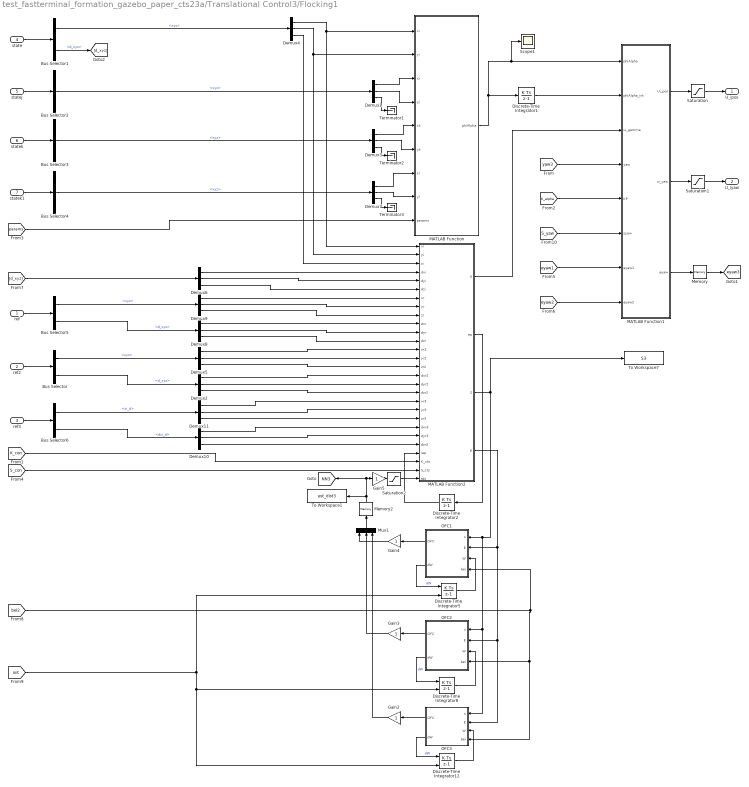
== system test_fastterminal_formation_gazebo_paper_cts23a/Translational Control3/Flocking1 ==
  ref : Inport
  ref2 : Inport  Port=2
  ref3 : Inport  Port=3
  state : Inport  Port=4
  statej : Inport  Port=5
  statek : Inport  Port=6
  statek1 : Inport  Port=7
  Bus Selector : BusSelector  OutputSignals=xyz,d_xyz
  Bus Selector1 : BusSelector  OutputSignals=xyz,d_xyz
  Bus Selector2 : BusSelector  OutputSignals=xyz
  Bus Selector3 : BusSelector  OutputSignals=xyz
  Bus Selector4 : BusSelector  OutputSignals=xyz
  Bus Selector5 : BusSelector  OutputSignals=xyz,d_xyz
  Bus Selector6 : BusSelector  OutputSignals=xi_d,dxi_d
  Demux{1..11} (11 alike) : Demux  Outputs=3
  Discrete-Time Integrator1 : DiscreteIntegrator  SampleTime=-1  LimitOutput=on  UpperSaturationLimit=5  LowerSaturationLimit=-5  ICPrevOutput=DiscIntNeverNeededParam  ICPrevScaledInput=DiscIntNeverNeededParam
  Discrete-Time Integrator12 : DiscreteIntegrator  InitialConditionSource=external  SampleTime=-1  UpperSaturationLimit=0.15  LowerSaturationLimit=-0.15  ICPrevOutput=DiscIntNeverNeededParam  ICPrevScaledInput=DiscIntNeverNeededParam
  Discrete-Time Integrator2 : DiscreteIntegrator  SampleTime=-1  LimitOutput=on  UpperSaturationLimit=2  LowerSaturationLimit=-2  ICPrevOutput=DiscIntNeverNeededParam  ICPrevScaledInput=DiscIntNeverNeededParam
  Discrete-Time Integrator5 : DiscreteIntegrator  InitialConditionSource=external  InitialCondition=0.25*ones(6,1)  SampleTime=-1  UpperSaturationLimit=0.15  LowerSaturationLimit=-0.15  ICPrevOutput=DiscIntNeverNeededParam  ICPrevScaledInput=DiscIntNeverNeededParam
  Discrete-Time Integrator8 : DiscreteIntegrator  InitialConditionSource=external  InitialCondition=0.25*ones(6,1)  SampleTime=-1  UpperSaturationLimit=0.15  LowerSaturationLimit=-0.15  ICPrevOutput=DiscIntNeverNeededParam  ICPrevScaledInput=DiscIntNeverNeededParam
  Gain{2..5} (4 alike) : Gain
  MATLAB Function : MATLAB Function  TreatAsAtomicUnit=on
  MATLAB Function1 : MATLAB Function  TreatAsAtomicUnit=on
  MATLAB Function2 : MATLAB Function  TreatAsAtomicUnit=on
  Memory : Memory
  Memory2 : Memory
  Mux1 : Mux  Inputs=3
  OFC1 : MATLAB Function  TreatAsAtomicUnit=on
  OFC2 : MATLAB Function  TreatAsAtomicUnit=on
  OFC3 : MATLAB Function  TreatAsAtomicUnit=on
  Saturation : Saturate  UpperLimit=1  LowerLimit=-1
  Saturation1 : Saturate  UpperLimit=1  LowerLimit=-1
  Saturation2 : Saturate  UpperLimit=0.9  LowerLimit=-0.9
  Scope1 : Scope
  Terminator1 : Terminator
  Terminator2 : Terminator
  Terminator3 : Terminator
  To Workspace1 : ToWorkspace  VariableName=est_dist3  SampleTime=-1
  To Workspace7 : ToWorkspace  VariableName=S3  SampleTime=-1
  U_ipos : Outport  VectorParamsAs1DForOutWhenUnconnected=off
  U_iyaw : Outport  Port=2  VectorParamsAs1DForOutWhenUnconnected=off
  tag scope: NN3=global, eyaw3=global
  wires:
  Saturation2/1 -> MATLAB Function2/28(NN)
  Demux2/1 -> MATLAB Function2/16(dxr2)
  Demux5/1 -> MATLAB Function2/13(xr2)
  Demux2/2 -> MATLAB Function2/17(dyr2)
  Demux5/2 -> MATLAB Function2/14(yr2)
  Demux2/3 -> MATLAB Function2/18(dzr2)
  Demux5/3 -> MATLAB Function2/15(zr2)
  Demux8/3 -> MATLAB Function2/12(dzr)
  Demux8/1 -> MATLAB Function2/10(dxr)
  Demux9/3 -> MATLAB Function2/9(zr)
  Demux9/1 -> MATLAB Function2/7(xr)
  Demux8/2 -> MATLAB Function2/11(dyr)
  Demux9/2 -> MATLAB Function2/8(yr)
  Bus Selector5/2 -> Demux8/1  "<d_xyz>"
  Bus Selector5/1 -> Demux9/1  "<xyz>"
  ref/1 -> Bus Selector5/1
  ref2/1 -> Bus Selector/1
  state/1 -> Bus Selector1/1
  Bus Selector/1 -> Demux5/1  "<xyz>"
  statej/1 -> Bus Selector2/1
  Bus Selector2/1 -> Demux1/1  "<xyz>"
  Demux4/1 -> MATLAB Function/1(xi), MATLAB Function2/1(xi)
  Demux4/2 -> MATLAB Function2/2(yi), MATLAB Function/2(yi)
  Demux1/1 -> MATLAB Function/3(xj)
  Demux1/2 -> MATLAB Function/4(yj)
  Discrete-Time Integrator1/1 -> MATLAB Function1/2(phiAlpha_int)
  MATLAB Function2/1(U) -> MATLAB Function1/3(ui_gamma)
  statek/1 -> Bus Selector3/1
  Demux3/1 -> MATLAB Function/5(xk)
  Demux3/2 -> MATLAB Function/6(yk)
  Bus Selector3/1 -> Demux3/1  "<xyz>"
  MATLAB Function/1(phiAlpha) -> Scope1/1, MATLAB Function1/1(phiAlpha), Discrete-Time Integrator1/1
  Demux4/3 -> MATLAB Function2/3(zi)
  Demux3/3 -> Terminator2/1
  MATLAB Function1/1(Ui_pos) -> Saturation/1
  Demux1/3 -> Terminator1/1
  statek1/1 -> Bus Selector4/1
  Demux7/1 -> MATLAB Function/7(xl)
  Demux7/2 -> MATLAB Function/8(yl)
  Demux7/3 -> Terminator3/1
  Bus Selector4/1 -> Demux7/1  "<xyz>"
  Bus Selector1/1 -> Demux4/1  "<xyz>"
  [yaw3] -> MATLAB Function1/4(yaw)
  MATLAB Function1/2(ui_yaw) -> Saturation1/1
  MATLAB Function2/2(ep) -> Discrete-Time Integrator2/1
  Discrete-Time Integrator2/1 -> MATLAB Function2/25(iep)
  [K_con] -> MATLAB Function2/26(K_cts)
  MATLAB Function1/3(eyaw) -> Memory/1
  [K_alpha] -> MATLAB Function1/5(KP)
  [params] -> MATLAB Function/9(params)
  [S_con] -> MATLAB Function2/27(S_cts)
  Bus Selector/2 -> Demux2/1  "<d_xyz>"
  [eyaw1] -> MATLAB Function1/7(eyaw1)
  [eyaw2] -> MATLAB Function1/8(eyaw2)
  Memory/1 -> [eyaw3]
  MATLAB Function2/3(S) -> OFC3/1(s), OFC2/1(s), OFC1/1(s), To Workspace7/1
  OFC3/1(OFC) -> Gain2/1
  OFC1/1(OFC) -> Gain4/1
  OFC2/1(OFC) -> Gain3/1
  OFC1/2(dW) -> Discrete-Time Integrator5/1  "dW"
  MATLAB Function2/4(E) -> OFC1/2(E), OFC3/2(E), OFC2/2(E)
  [bel2] -> OFC3/4(bel), OFC2/4(bel), OFC1/4(bel)
  [init] -> Discrete-Time Integrator12/2, Discrete-Time Integrator8/2, Discrete-Time Integrator5/2
  OFC3/2(dW) -> Discrete-Time Integrator12/1  "dW"
  Discrete-Time Integrator12/1 -> OFC3/3(W)
  Gain3/1 -> Mux1/2
  Discrete-Time Integrator8/1 -> OFC2/3(W)
  Gain2/1 -> Mux1/3
  OFC2/2(dW) -> Discrete-Time Integrator8/1  "dW"
  Gain4/1 -> Mux1/1
  Memory2/1 -> Gain5/1, [NN3], To Workspace1/1
  Saturation/1 -> U_ipos/1
  Saturation1/1 -> U_iyaw/1
  Discrete-Time Integrator5/1 -> OFC1/3(W)
  Mux1/1 -> Memory2/1
  Bus Selector1/2 -> [d_xyz]  "<d_xyz>"
  Demux6/1 -> MATLAB Function2/4(dxi)
  Demux6/2 -> MATLAB Function2/5(dyi)
  Demux6/3 -> MATLAB Function2/6(dzi)
  [d_xyz] -> Demux6/1
  Gain5/1 -> Saturation2/1
  Bus Selector6/2 -> Demux10/1  "<dxi_d>"
  Bus Selector6/1 -> Demux11/1  "<xi_d>"
  ref3/1 -> Bus Selector6/1
  Demux11/3 -> MATLAB Function2/21(zr3)
  Demux10/3 -> MATLAB Function2/24(dzr3)
  Demux11/2 -> MATLAB Function2/20(yr3)
  Demux10/2 -> MATLAB Function2/23(dyr3)
  Demux11/1 -> MATLAB Function2/19(xr3)
  Demux10/1 -> MATLAB Function2/22(dxr3)
  [S_yaw] -> MATLAB Function1/6(syaw)

== matlab function test_fastterminal_formation_gazebo_paper_cts23a/Translational Control1/Flocking1/OFC1 ==
  settings: updateMethod=DISCRETE  sampleTime=0.05
  data: OFC output size=1; dW output; s input; E input; W input; bel input
function [OFC,dW] = fcn(s, E,W, bel)

m = 70;
sigma = bel(1); %12
alpha_ofc = bel(2); %1
r1 = bel(3);
r2 = bel(4);

%Sliding
sx = s(1,1);

ex = E(1,1);
dex = E(4,1);

persistent phivec

if isempty(phivec)
    phivec = zeros(m,1);
end

mu1 = linspace(-r1, r1, m); 
mu2 = linspace(-r2, r2, m); 

for i = 1:1:m
    phivec(i) = exp(-(norm(ex-mu1(i))^2+norm(dex-mu2(i))^2)/(sigma^2));
end

OFC = W'*phivec;

dW = -alpha_ofc*sx*phivec;

== matlab function test_fastterminal_formation_gazebo_paper_cts23a/Virtual_leader ==
  data: t input; xi_d output; dxi_d output; Xd input; f input
function [xi_d, dxi_d]  = fcn(t, Xd, f)
%#codegen



%f=1/100;    %freq in Hz
radius= 0.275;   %radius in meters 0.15
sel=1;      %inputs or parameters dont work! only local vars ...

if sel == 1
    if t < 30
       xd     =  0;
       xdotd  =  0;
           
       yd     = 0;
       ydotd  = 0;
           
       zd     = 1;  
       zdotd  = 0; 
           
       xi_d =[xd; yd; zd];
       dxi_d=[xdotd; ydotd; zdotd]; 
       
    % elseif t < 70
    %     xd     =  0.4;
    %     xdotd  =  0;
    % 
    %     yd     = -0.4;
    %     ydotd  = 0;
    % 
    %     zd     = 2.5;  
    %     zdotd  = 0; 
    % 
    %     xi_d =[xd; yd; zd];
    %     dxi_d=[xdotd; ydotd; zdotd]; 
        
    elseif t < 120  %140
       xd     = 0.1 + radius*sin(2*pi*f*t);
       xdotd  = radius*2*pi*f*cos(2*pi*f*t);
            
       yd     = 0.15 + radius*cos(2*pi*f*t);
       ydotd  = -radius*2*pi*f*sin(2*pi*f*t);
            
       zd     = 1.2; %0.2*cos(2*pi*f*t) + 1;
       zdotd  = 0; %-0.2*2*pi*f*sin(2*pi*f*t);
           
       xi_d =[xd; yd; zd];
       dxi_d=[xdotd; ydotd; zdotd];
    else
        xd     =  -0.2;
        xdotd  =  0;
            
        yd     = 0.1;
        ydotd  = 0;
            
        zd     = 1.1;  
        zdotd  = 0; 
            
        xi_d =[xd; yd; zd];
        dxi_d=[xdotd; ydotd; zdotd];        
    end
end

 if(sel==2)
     xd     =  Xd(1);
     xdotd  =  0;
          
     yd     = Xd(2);
     ydotd  = 0;
          
     zd     = Xd(3);  
     zdotd  = 0; 
          
     xi_d =[xd; yd; zd];
     dxi_d=[xdotd; ydotd; zdotd]; 
     
 end

== matlab function test_fastterminal_formation_gazebo_paper_cts23a/Translational Control2/Flocking1/MATLAB Function ==
  data: xi input; yi input; phiAlpha output; xj input; yj input; xk input; yk input; xl input; yl input; params input

function phiAlpha  = phiAlphaFcn(xi, yi, xj, yj, xk, yk, xl, yl, params)
    
    % Flocking parameters
    epsilon = params(1); a = params(2); b = params(3); c = params(4); d = params(5); h = params(6);

    e = abs(a - b) / sqrt(4*a*b) ;

    cAlpha = sigmaNormFun(c, epsilon) ;
    dAlpha = sigmaNormFun(d, epsilon) ;

    %%
    Pi = [xi;yi] ;
    Pj = [xj;yj] ;
    Pk = [xk;yk] ;
    Pl = [xl;yl] ;

    %%
    sigmaNormj = sigmaNormFun(Pj - Pi, epsilon) ;
    nij = gradSigmaFun(Pj - Pi, epsilon) ;
    
    sigmaNormk = sigmaNormFun(Pk - Pi, epsilon) ;
    nik = gradSigmaFun(Pk - Pi, epsilon) ;

    sigmaNorml = sigmaNormFun(Pl - Pi, epsilon) ;
    nil = gradSigmaFun(Pl - Pi, epsilon) ;

    %%
    sigma1j = sigma1Fun(sigmaNormj - dAlpha + e) ;
    sigma1k = sigma1Fun(sigmaNormk - dAlpha + e) ;
    sigma1l = sigma1Fun(sigmaNorml - dAlpha + e) ;
            
    %% Position
    phiAlphaj = 0.5 * bumpFcn(sigmaNormj/cAlpha,h) * ((a+b)*sigma1j + (a-b)) ;
    phiAlphanij = phiAlphaj.* nij ;
    
    phiAlphak = 0.5 * bumpFcn(sigmaNormk/cAlpha,h) * ((a+b)*sigma1k + (a-b)) ;
    phiAlphanik = phiAlphak.* nik ;

    phiAlphal = 0.5 * bumpFcn(sigmaNorml/cAlpha,h) * ((a+b)*sigma1l + (a-b)) ;
    phiAlphanil = phiAlphal.* nil ;

    phiAlpha = phiAlphanij + phiAlphanik + phiAlphanil;

    
end

== matlab function test_fastterminal_formation_gazebo_paper_cts23a/Translational Control2/Flocking1/MATLAB Function1 ==
  data: phiAlpha input; phiAlpha_int input; ui_gamma input; yaw input; Ui_pos output size=3; ui_yaw output; KP input; syaw input; eyaw output; eyaw1 input; eyaw3 input

function [Ui_pos, ui_yaw, eyaw]  = ctrlLaw(phiAlpha, phiAlpha_int, ui_gamma, yaw, KP, syaw, eyaw1, eyaw3)  
    
    % Control gains and parameters
    k1 = syaw(1); sigma = syaw(2); beta = syaw(3); 
    ks = syaw(4); ke = syaw(5);

    % Control gains and parameters
    Kx = KP(1); Ky = KP(2); Kz = KP(3);
    Kix = KP(4); Kiy = KP(5); Kiz = KP(6);
    Kyaw = KP(7); Kdyaw = KP(8); Kiyaw = KP(9);
    offset = KP(10);
    
    eyaw = 0 - yaw(1);
    deyaw = 0 - yaw(2);

    %Manifold
    Syaw = manifold_ter_back_yaw(eyaw, deyaw, sigma, beta);
    %Control
    ui_yaw = back_ter_yaw_con(eyaw, Syaw, sigma, beta, k1, ks, ke);
    hz_dot = ui_gamma(3,1);  %

    if eyaw < offset && eyaw > -offset && eyaw1 < offset && eyaw1 > -offset && eyaw3 < offset && eyaw3 > -offset 
        hx_dot =  ui_gamma(1,1);  %Kx * phiAlpha(1,1) + Kix * phiAlpha_int(1,1) + 
        hy_dot =  ui_gamma(2,1);  %Ky * phiAlpha(2,1) + Kiy * phiAlpha_int(2,1) + 
    else
        hx_dot =  0;  %
        hy_dot =  0;  %
    end    

    Ui_pos = [hx_dot; hy_dot; hz_dot] ;
    

end

== matlab function test_fastterminal_formation_gazebo_paper_cts23a/Translational Control2/Flocking1/MATLAB Function2 ==
  data: xi input; yi input; zi input; dxi input; dyi input; dzi input; U output; xr input; yr input; zr input; dxr input; dyr input; dzr input; xr2 input; yr2 input; zr2 input; dxr2 input; dyr2 input; dzr2 input; iep input size=3; ep output size=3; S output; E output; K_cts input; S_cts input; NN input

function [U, ep, S, E] = naviFeedback(xi, yi, zi, dxi, dyi, dzi, xr, yr, zr, dxr, dyr, dzr, xr2, yr2, zr2, dxr2, dyr2, dzr2, iep, K_cts, S_cts, NN)
    
    Kp = K_cts(1); Kpz = K_cts(2);

    % Cts manifold
    C1_xy = S_cts(1); C2_xy = S_cts(2); alpha1_xy = S_cts(3); alpha2_xy = S_cts(4);
    C1_z = S_cts(5); C2_z = S_cts(6); alpha1_z = S_cts(7); alpha2_z = S_cts(8);
    
    %errors
    ex = (xr - xi - 0.75) + (xr2 - xi - 0.25);
    ey = (yr - yi - 0.43) + (yr2 - yi - 0.43);
    ez = (zr - zi) + (zr2 - zi);
    ep = [ex;ey;ez];

    dex = (dxr - dxi) + (dxr2 - dxi);
    dey = (dyr - dyi) + (dyr2 - dyi);
    dez = (dzr - dzi) + (dzr2 - dzi);
    E = [ex;ey;ez;dex;dey;dez];

    %error integrals
    iex = iep(1);
    iey = iep(2);
    iez = iep(3);
    
    %Manifold definitions
    Sx = manifold_pos_int(iex, ex, C1_xy, C2_xy, alpha1_xy, alpha2_xy);
    Sy = manifold_pos_int(iey, ey, C1_xy, C2_xy, alpha1_xy, alpha2_xy);
    Sz = manifold_pos_int(iez, ez, C1_z, C2_z, alpha1_z, alpha2_z);

    S = [Sx;Sy;Sz];

    ux = fast_con2(iex, ex, Sx, dxr + dxr2, C1_xy, C2_xy, alpha1_xy, alpha2_xy, Kp) - NN(1);
    uy = fast_con2(iey, ey, Sy, dyr + dyr2, C1_xy, C2_xy, alpha1_xy, alpha2_xy, Kp) - NN(2);
    uz = fast_con2(iez, ez, Sz, dzr + dzr2, C1_z, C2_z, alpha1_z, alpha2_z, Kpz) - NN(3);

    U = [ux;uy;uz];
end

== matlab function test_fastterminal_formation_gazebo_paper_cts23a/Translational Control1/Flocking1/OFC2 ==
  settings: updateMethod=DISCRETE  sampleTime=0.05
  data: OFC output size=1; dW output; s input; E input; W input; bel input
function [OFC,dW] = fcn(s, E,W, bel)

m = 70;
sigma = bel(1); %12
alpha_ofc = bel(2); %1
r1 = bel(3);
r2 = bel(4);

%Sliding
sy = s(2,1);

ey = E(2,1);
dey = E(5,1);

persistent phivec

if isempty(phivec)
    phivec = zeros(m,1);
end

mu1 = linspace(-r1, r1, m);
mu2 = linspace(-r2, r2, m);

for i = 1:1:m
    phivec(i) = exp(-(norm(ey-mu1(i))^2+norm(dey-mu2(i))^2)/(sigma^2));
end

OFC = W'*phivec;

dW = -alpha_ofc*sy*phivec;

== matlab function test_fastterminal_formation_gazebo_paper_cts23a/Translational Control1/Flocking1/OFC3 ==
  settings: updateMethod=DISCRETE  sampleTime=0.05
  data: OFC output size=1; dW output; s input; E input; W input; bel input
function [OFC,dW] = fcn(s, E, W, bel)

m = 70;
sigma = bel(5); %12
alpha_ofc = bel(6); %1
r1 = bel(7);
r2 = bel(8);

%Sliding
sz = s(3,1);

ez = E(3,1);
dez = E(6,1);

persistent phivec

if isempty(phivec)
    phivec = zeros(m,1);
end

mu1 = linspace(-r1, r1, m); 
mu2 = linspace(-r2, r2, m); 

for i = 1:1:m
    phivec(i) = exp(-(norm(ez-mu1(i))^2+norm(dez-mu2(i))^2)/(sigma^2));
end

OFC = W'*phivec;

dW = -alpha_ofc*sz*phivec;

== matlab function test_fastterminal_formation_gazebo_paper_cts23a/Translational Control3/Flocking1/MATLAB Function ==
  data: xi input; yi input; phiAlpha output; xj input; yj input; xk input; yk input; xl input; yl input; params input

function phiAlpha  = phiAlphaFcn(xi, yi, xj, yj, xk, yk, xl, yl, params)
    
    % Flocking parameters
    epsilon = params(1); a = params(2); b = params(3); c = params(4); d = params(5); h = params(6);

    e = abs(a - b) / sqrt(4*a*b) ;

    cAlpha = sigmaNormFun(c, epsilon) ;
    dAlpha = sigmaNormFun(d, epsilon) ;

    %%
    Pi = [xi;yi] ;
    Pj = [xj;yj] ;
    Pk = [xk;yk] ;
    Pl = [xl;yl] ;

    %%
    sigmaNormj = sigmaNormFun(Pj - Pi, epsilon) ;
    nij = gradSigmaFun(Pj - Pi, epsilon) ;
    
    sigmaNormk = sigmaNormFun(Pk - Pi, epsilon) ;
    nik = gradSigmaFun(Pk - Pi, epsilon) ;

    sigmaNorml = sigmaNormFun(Pl - Pi, epsilon) ;
    nil = gradSigmaFun(Pl - Pi, epsilon) ;

    %%
    sigma1j = sigma1Fun(sigmaNormj - dAlpha + e) ;
    sigma1k = sigma1Fun(sigmaNormk - dAlpha + e) ;
    sigma1l = sigma1Fun(sigmaNorml - dAlpha + e) ;
            
    %% Position
    phiAlphaj = 0.5 * bumpFcn(sigmaNormj/cAlpha,h) * ((a+b)*sigma1j + (a-b)) ;
    phiAlphanij = phiAlphaj.* nij ;
    
    phiAlphak = 0.5 * bumpFcn(sigmaNormk/cAlpha,h) * ((a+b)*sigma1k + (a-b)) ;
    phiAlphanik = phiAlphak.* nik ;

    phiAlphal = 0.5 * bumpFcn(sigmaNorml/cAlpha,h) * ((a+b)*sigma1l + (a-b)) ;
    phiAlphanil = phiAlphal.* nil ;

    phiAlpha = phiAlphanij + phiAlphanik + phiAlphanil;

    
end

== matlab function test_fastterminal_formation_gazebo_paper_cts23a/Translational Control3/Flocking1/MATLAB Function1 ==
  data: phiAlpha input; phiAlpha_int input; ui_gamma input; yaw input; Ui_pos output size=3; ui_yaw output; KP input; syaw input; eyaw output; eyaw1 input; eyaw2 input

function [Ui_pos, ui_yaw, eyaw]  = ctrlLaw(phiAlpha, phiAlpha_int, ui_gamma, yaw, KP, syaw, eyaw1, eyaw2)  
    
    % Control gains and parameters
    k1 = syaw(1); sigma = syaw(2); beta = syaw(3); 
    ks = syaw(4); ke = syaw(5);

    % Control gains and parameters
    Kx = KP(1); Ky = KP(2); Kz = KP(3);
    Kix = KP(4); Kiy = KP(5); Kiz = KP(6);
    Kyaw = KP(7); Kdyaw = KP(8); Kiyaw = KP(9);
    offset = KP(10);
    
    eyaw = 0 - yaw(1);
    deyaw = 0 - yaw(2);

    %Manifold
    Syaw = manifold_ter_back_yaw(eyaw, deyaw, sigma, beta);
    %Control
    ui_yaw = back_ter_yaw_con(eyaw, Syaw, sigma, beta, k1, ks, ke);
    hz_dot = ui_gamma(3,1);  %

    if eyaw < offset && eyaw > -offset && eyaw1 < offset && eyaw1 > -offset && eyaw2 < offset && eyaw2 > -offset 
        hx_dot =  ui_gamma(1,1);  %Kx * phiAlpha(1,1) + Kix * phiAlpha_int(1,1) + 
        hy_dot =  ui_gamma(2,1);  %Ky * phiAlpha(2,1) + Kiy * phiAlpha_int(2,1) + 
    else
        hx_dot =  0;  %
        hy_dot =  0;  %
    end    

    Ui_pos = [hx_dot; hy_dot; hz_dot] ;
    

end
